simulink subsystem "Thrust_Tables"  (R2024a)
settings: Solver=VariableStepAuto  StartTime=0.0  StopTime=10.0  RelTol=1e-3
undefined symbols (not defined in the file): Rocket
settings Model: Creator=Andrew Radulovich  LastModifiedBy=thatf
settings ModelReferenceCC: EnableRefExpFcnMdlSchedulingChecks=on
settings RTWCC: GPUComputeCapability=3.5

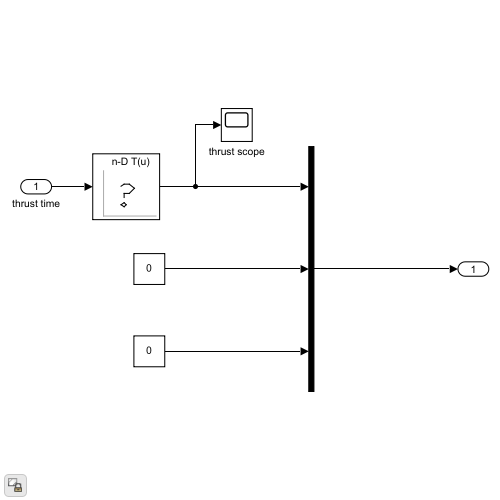
[thumbnail: Simulink's stored preview of the top-level diagram]
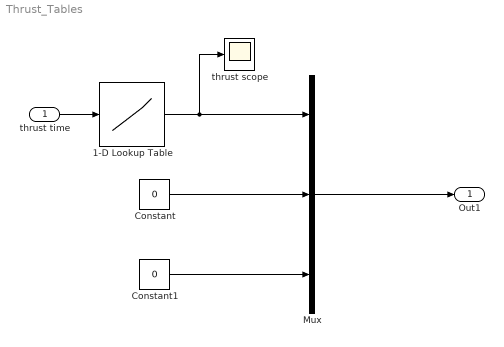
== system Thrust_Tables ==
  thrust time : Inport
  1-D Lookup Table : Lookup_n-D  NumberOfTableDimensions=1  BreakpointsForDimension1=Rocket.Tx(:,1)  IndexSearchMethod=Linear search  BeginIndexSearchUsingPreviousIndexResult=on  Table=Rocket.Tx(:,2)  ExtrapMethod=Clip  UseLastTableValue=on  InternalRulePriority=Speed  RndMeth=Simplest
  Constant : Constant  Value=0
  Constant1 : Constant  Value=0
  Mux : Mux  Inputs=3
  thrust scope : Scope
  Out1 : Outport
  wires:
  1-D Lookup Table/1 -> thrust scope/1, Mux/1
  Constant/1 -> Mux/2
  Constant1/1 -> Mux/3
  Mux/1 -> Out1/1
  thrust time/1 -> 1-D Lookup Table/1
